simulink model "assigment3_3_2"  (R2022b)
settings: Solver=FixedStepAuto  StartTime=0.0  StopTime=500  FixedStep=0.001  RelTol=1e-3
settings Model: Creator=iran sistem  LastModifiedBy=iran sistem

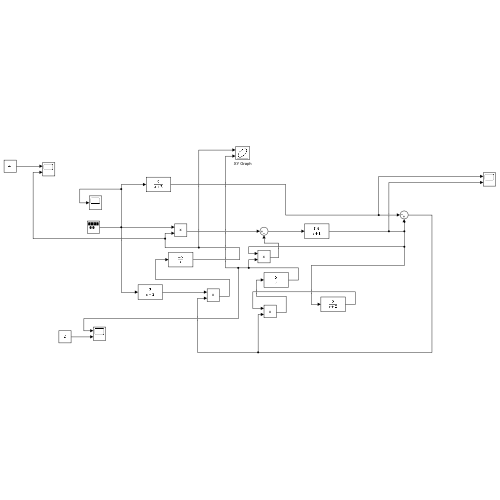
[thumbnail: Simulink's stored preview of the top-level diagram]
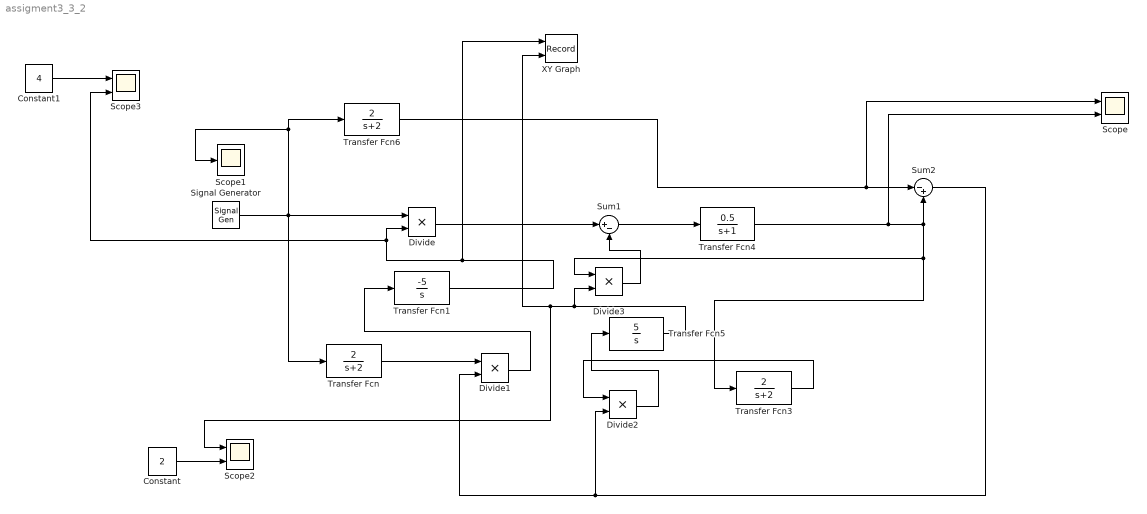
== system assigment3_3_2 ==
  Constant : Constant  Value=2
  Constant1 : Constant  Value=4
  Divide{,1..3} (4 alike) : Product  Inputs=**
  Scope : Scope  NumInputPorts=2
  Scope1 : Scope
  Scope2 : Scope  NumInputPorts=2
  Scope3 : Scope  NumInputPorts=2
  Signal Generator : SignalGenerator  WaveForm=square  Units=rad/sec
  Sum1 : Sum  Inputs=|+-
  Sum2 : Sum  Inputs=|-+
  Transfer Fcn : TransferFcn  Numerator=[2]  Denominator=[1 2]
  Transfer Fcn1 : TransferFcn  Numerator=[-5]  Denominator=[1 0]
  Transfer Fcn3 : TransferFcn  Numerator=[2]  Denominator=[1 2]
  Transfer Fcn4 : TransferFcn  Numerator=[0.5]  Denominator=[1 1]
  Transfer Fcn5 : TransferFcn  Numerator=[5]  Denominator=[1 0]
  Transfer Fcn6 : TransferFcn  Numerator=[2]  Denominator=[1 2]
  XY Graph : Record  FileSettingsInternal="{\"entries\":[{\"content\":{\"excelSettings\":{\"content\":{},\"type\":\"Streamout.ExcelSettings\"}},\"type\":\"Streamout.FileSettingStorage\",\"uuid\":\"d05fe701-2dbf-48ef-a8fb-f138c140f14e\"}],\"packageUris\":[\"http://schema.mathworks.com/mf0/streamout_blocks/R2020a\"],\"version\":\"1.0\"}"  Layout=[1 1]  SignalsInternal="{\"entries\":[{\"content\":{\"signals\":[{\"content\":{\"blockPath\":[\"untitled/XY Graph\"],\"channel\":[],\"dimensions\":[1],\"domain\":\"untitled/XY Graph\",\"lineColor\":\"#a2142f\",\"plots\":[1],\"port\":1,\"sid\":[\"\"],\"signalID\":32734,\"signalName\":\"Transfer Fcn1\"},\"type\":\"RecordBlkView.Signal\",\"uuid\":\"46359e6f-5e17-467c-a9f7-fc2fc9c7e7fd\"},{\"content\":{\"blockPath\":[\"untitled/XY Graph\"],\"channel\":[],\"dimensions\":[1],\"domain\":\"untitled/XY Graph\",\"lineColor\":\"#139fff\",\"plots\":[1],\"port\":2,\"sid\":[\"\"],\"signalID\":32738,\"signalName\":\"Transfer Fcn5\"},\"type\":\"RecordBlkView.Signal\",\"uuid\":\"7fe0e64c-34af-415a-ba34-b893dd400546\"}]},\"type\":\"RecordBlkView.InputSignals\",\"uuid\":\"eb678516-cfff-4d57-bd7a-74c783486aae\"}],\"packageUris\":[\"http://schema.mathworks.com/mf0/streamout_blocks/R2020a\"],\"version\":\"1.0\"}"  VisualizationBindings="{\"xyplotplugin\":{\"info\":[{\"series\":[{\"bindingParametersList\":[{\"parameter\":\"X-Axis\",\"signalID\":32734,\"signalName\":\"Transfer Fcn1\"},{\"parameter\":\"Y-Axis\",\"signalID\":32738,\"signalName\":\"Transfer Fcn5\"}],\"seriesID\":7161}],\"subplotID\":1}]}}"  CompatibilityTag=XY
  wires:
  Transfer Fcn/1 -> Divide1/1
  Transfer Fcn1/1 -> XY Graph/1, Scope3/2, Divide/2
  Divide1/1 -> Transfer Fcn1/1
  Divide/1 -> Sum1/1
  Divide2/1 -> Transfer Fcn5/1
  Transfer Fcn5/1 -> XY Graph/2, Scope2/1, Divide3/2
  Divide3/1 -> Sum1/2
  Sum1/1 -> Transfer Fcn4/1
  Transfer Fcn3/1 -> Divide2/1
  Transfer Fcn6/1 -> Scope/1, Sum2/1
  Transfer Fcn4/1 -> Scope/2, Divide3/1, Transfer Fcn3/1, Sum2/2
  Sum2/1 -> Divide2/2, Divide1/2
  Constant/1 -> Scope2/2
  Constant1/1 -> Scope3/1
  Signal Generator/1 -> Transfer Fcn/1, Scope1/1, Transfer Fcn6/1, Divide/1
